simulink library "SimControllerFcns"  (R2014b)
settings: Solver=ode45  StartTime=0.0  StopTime=10.0  RelTol=1e-3
undefined symbols (not defined in the file): K, wheel
settings Model: Creator=scastro  LastModifiedBy=scastro

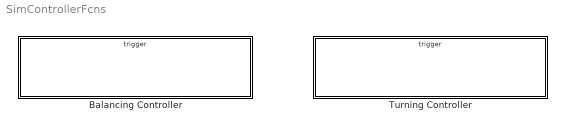
== system SimControllerFcns ==
  Balancing Controller : Subsystem  TreatAsAtomicUnit=on
  Turning Controller : Subsystem  TreatAsAtomicUnit=on

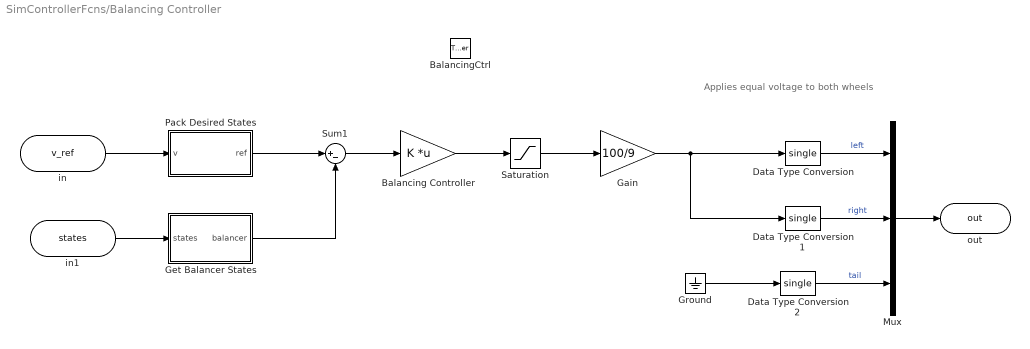
== system SimControllerFcns/Balancing Controller ==
  note: Applies equal voltage to both wheels
  BalancingCtrl : TriggerPort  TriggerType=function-call  IsSimulinkFunction=on  FunctionName=BalancingCtrl
  Balancing Controller : Gain  Gain=K  Multiplication=Matrix(K*u)
  Data Type Conversion : DataTypeConversion  OutDataTypeStr=single
  Data Type Conversion1 : DataTypeConversion  OutDataTypeStr=single
  Data Type Conversion2 : DataTypeConversion  OutDataTypeStr=single
  Gain : Gain  Gain=100/9
  Get Balancer States : Subsystem
  Ground : Ground
  Mux : Mux  Inputs=3
  Pack Desired States : Subsystem
  Saturation : Saturate  UpperLimit=9  LowerLimit=-9  OutDataTypeStr=single
  Sum1 : Sum  Inputs=|+-
  in : ArgIn  OutDataTypeStr=single  ArgumentName=v_ref
  in1 : ArgIn  Port=2  OutDataTypeStr=Bus: States_Bus  ArgumentName=states
  out : ArgOut  OutDataTypeStr=single  PortDimensions=3  ArgumentName=out
  wires:
  Balancing Controller/1 -> Saturation/1
  Sum1/1 -> Balancing Controller/1
  Pack Desired States/1(ref) -> Sum1/1
  in/1 -> Pack Desired States/1(v)
  Ground/1 -> Data Type Conversion2/1
  Mux/1 -> out/1
  Data Type Conversion/1 -> Mux/1  "left"
  Data Type Conversion1/1 -> Mux/2  "right"
  Data Type Conversion2/1 -> Mux/3  "tail"
  Gain/1 -> Data Type Conversion1/1, Data Type Conversion/1
  Saturation/1 -> Gain/1
  in1/1 -> Get Balancer States/1(states)
  Get Balancer States/1(balancer) -> Sum1/2

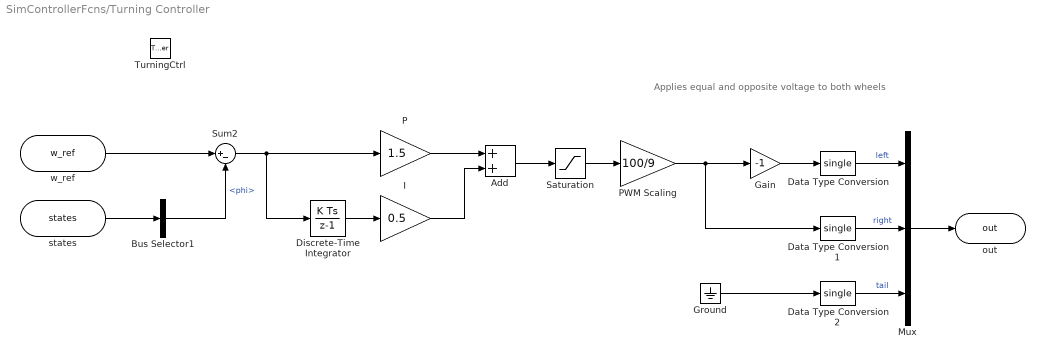
== system SimControllerFcns/Turning Controller ==
  note: Applies equal and opposite voltage to both wheels
  TurningCtrl : TriggerPort  TriggerType=function-call  IsSimulinkFunction=on  FunctionName=TurningCtrl
  Add : Sum
  Bus Selector1 : BusSelector  OutputSignals=phi
  Data Type Conversion : DataTypeConversion  OutDataTypeStr=single
  Data Type Conversion1 : DataTypeConversion  OutDataTypeStr=single
  Data Type Conversion2 : DataTypeConversion  OutDataTypeStr=single
  Discrete-Time Integrator : DiscreteIntegrator  SampleTime=-1
  Gain : Gain  Gain=-1
  Ground : Ground
  I : Gain  Gain=0.5
  Mux : Mux  Inputs=3
  P : Gain  Gain=1.5
  PWM Scaling : Gain  Gain=100/9
  Saturation : Saturate  UpperLimit=2  LowerLimit=-2
  Sum2 : Sum  Inputs=|+-
  w_ref : ArgIn  OutDataTypeStr=single  ArgumentName=w_ref
  states : ArgIn  Port=2  OutDataTypeStr=Bus: States_Bus  ArgumentName=states
  out : ArgOut  OutDataTypeStr=single  PortDimensions=3  ArgumentName=out
  wires:
  PWM Scaling/1 -> Data Type Conversion1/1, Gain/1
  Data Type Conversion2/1 -> Mux/3  "tail"
  Data Type Conversion1/1 -> Mux/2  "right"
  Data Type Conversion/1 -> Mux/1  "left"
  Ground/1 -> Data Type Conversion2/1
  P/1 -> Add/1
  Bus Selector1/1 -> Sum2/2  "<phi>"
  Sum2/1 -> Discrete-Time Integrator/1, P/1
  Gain/1 -> Data Type Conversion/1
  states/1 -> Bus Selector1/1
  w_ref/1 -> Sum2/1
  Mux/1 -> out/1
  Add/1 -> Saturation/1
  I/1 -> Add/2
  Discrete-Time Integrator/1 -> I/1
  Saturation/1 -> PWM Scaling/1

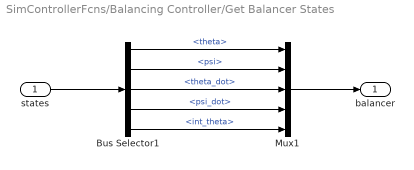
== system SimControllerFcns/Balancing Controller/Get Balancer States ==
  states : Inport
  Bus Selector1 : BusSelector  OutputSignals=balancerStates.theta,balancerStates.psi,balancerStates.theta_dot,balancerStates.psi_dot,balancerStates.int_theta
  Mux1 : Mux  Inputs=5
  balancer : Outport
  wires:
  Bus Selector1/1 -> Mux1/1  "<theta>"
  states/1 -> Bus Selector1/1
  Mux1/1 -> balancer/1
  Bus Selector1/2 -> Mux1/2  "<psi>"
  Bus Selector1/4 -> Mux1/4  "<psi_dot>"
  Bus Selector1/3 -> Mux1/3  "<theta_dot>"
  Bus Selector1/5 -> Mux1/5  "<int_theta>"

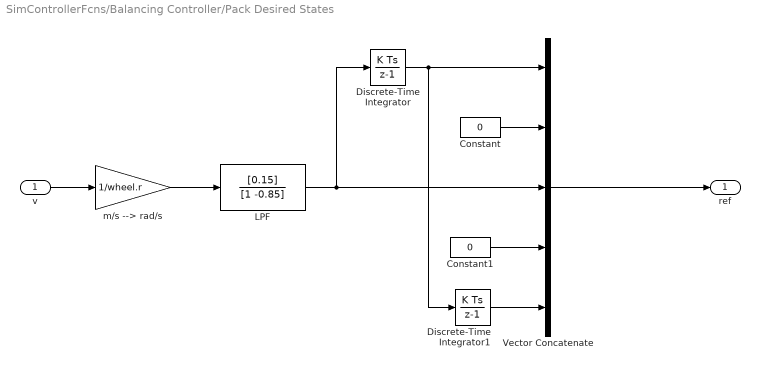
== system SimControllerFcns/Balancing Controller/Pack Desired States ==
  v : Inport
  Constant : Constant  Value=0  OutDataTypeStr=single
  Constant1 : Constant  Value=0  OutDataTypeStr=single
  Discrete-Time Integrator : DiscreteIntegrator  SampleTime=-1
  Discrete-Time Integrator1 : DiscreteIntegrator  SampleTime=-1
  LPF : DiscreteFilter  Numerator=[0.15]  Denominator=[1 -0.85]
  Vector Concatenate : Concatenate  NumInputs=5
  m/s --> rad/s : Gain  Gain=1/wheel.r
  ref : Outport
  wires:
  Vector Concatenate/1 -> ref/1
  Discrete-Time Integrator/1 -> Vector Concatenate/1, Discrete-Time Integrator1/1
  Constant1/1 -> Vector Concatenate/4
  m/s --> rad/s/1 -> LPF/1
  Constant/1 -> Vector Concatenate/2
  v/1 -> m/s --> rad/s/1
  Discrete-Time Integrator1/1 -> Vector Concatenate/5
  LPF/1 -> Discrete-Time Integrator/1, Vector Concatenate/3
